simulink model "manifold_pressure"  (R2018a)
settings: Solver=ode45  StartTime=0.0  StopTime=10.0  RelTol=1e-3  EnableMultiTasking=on
PreLoadFcn:
  | load manifold_pressure;
  | 
  | u = [mdot_in, w];
values from neighbouring files (symbols this model uses):
  mdot_in = [10.1509376684 10.1509376668 10.1509376591 10.1509376202 10.1509374255 10.1509364481 10.150931462 10.1509113235 10.1509113235 10.1508812304 10.1508812105 10.1508812105 ... (2511 elements, 2511x1)]    [manifold_press_start.mat]    (also in manifold_pressure.mat)
  w = [209.48 209.479999353 209.479996118 209.479979943 209.479899069 209.47949471 209.477473188 209.469890596 209.469890596 209.459798509 209.459792207 209.459792207 ... (2511 elements, 2511x1)]    [manifold_press_start.mat]    (also in manifold_pressure.mat)
settings Model: Creator=nicholas  LastModifiedBy=bneiswan
settings DataIOCC: LimitDataPoints=on  LoadExternalInput=on  SaveFormat=Array  SignalLoggingName=sigsOut
settings OptimizationCC: ExpressionDepthLimit=2147483647  InitFltsAndDblsToZero=on  LifeSpan=inf
settings DebuggingCC: SaveWithParameterizedLinksMsg=none  UnderspecifiedInitializationDetection=Classic  MergeDetectMultiDrivingBlocksExec=none  SignalResolutionControl=TryResolveAllWithWarning  MultiTaskDSMMsg=warning  MultiTaskCondExecSysMsg=none  ParameterPrecisionLossMsg=none  FcnCallInpInsideContextMsg=warning  AllowSymbolicDim=off  StateNameClashWarn=warning  SFUnexpectedBacktrackingDiag=warning  SFNoUnconditionalDefaultTransitionDiag=warning  SFExecutionAtInitializationDiag=none
settings HardwareCC: ProdBitPerPointer=32  ProdBitPerSizeT=32  ProdBitPerPtrDiffT=32  ProdLargestAtomicFloat=None  ProdIntDivRoundTo=Undefined  ProdEndianess=Unspecified  ProdWordSize=32  ProdHWDeviceType=32-bit Generic  TargetUnknown=on
settings ModelReferenceCC: PropagateSignalLabelsOutOfModel=off
settings CodeAppCC: StateflowObjectComments=on
settings GRTTargetCC: TargetFcnLib=ansi_tfl_tmw.mat  TargetLangStandard=C89/C90 (ANSI)  GeneratePreprocessorConditionals=Disable all  CombineOutputUpdateFcns=off  GRTInterface=on
settings ConfigComp: CovMetricSettings=dw  CovHtmlReporting=on  CovSaveCumulativeToWorkspaceVar=on  CovSaveSingleToWorkspaceVar=on  CovExternalEMLEnable=off  CovSFcnEnable=off

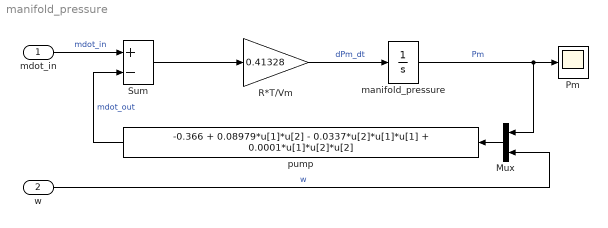
== system manifold_pressure ==
  mdot_in : Inport
  w : Inport  Port=2
  Mux : Mux  Inputs=2
  Pm : Scope
  R*T/Vm : Gain  Gain=0.41328  SaturateOnIntegerOverflow=on  OutDataTypeStr=Inherit: Same as input  ParamDataTypeStr=Inherit: Same as input
  Sum : Sum  Inputs=+-  SaturateOnIntegerOverflow=on  InputSameDT=on  OutDataTypeStr=Inherit: Same as first input
  manifold_pressure : Integrator  InitialCondition=0.543
      settings: AttributesFormatString=p0 = %<InitialCondition>\n\n
  pump : Fcn  Expr=-0.366 + 0.08979*u[1]*u[2] - 0.0337*u[2]*u[1]*u[1] + 0.0001*u[1]*u[2]*u[2]
  wires:
  Sum/1 -> R*T/Vm/1
  Mux/1 -> pump/1
  R*T/Vm/1 -> manifold_pressure/1  "dPm_dt"
  w/1 -> Mux/2  "w"
  manifold_pressure/1 -> Mux/1, Pm/1  "Pm"
  mdot_in/1 -> Sum/1  "mdot_in"
  pump/1 -> Sum/2  "mdot_out"
